simulink model "NeuromuscularModelwReflex2"  (R2019b)
settings: Solver=ode15s  StartTime=0.0  StopTime=30  MaxStep=.01  RelTol=1e-4  AbsTol=1e-6  EnableMultiTasking=on
values from neighbouring files (symbols this model uses):
  dt_visual = 1/30    (= 0.0333333333333)    [evaluateCost.m]    (also in optimize.m)
  LceOffsetTA = 1-0.5*w    [ControlParams.m]
  legAngleTgt = 1.2    [ControlParams.m]    (also in assignGains_novirtmuscle.m = Gains(38))
  LlegLengthClr = .9    (= 0.9)    [ControlParams.m]    (also in assignGains.m = Gains(39); assignGains_novirtmuscle.m = Gains(20))
  LongDelay = 0.020    (= 0.02)    [ControlParams.m]
  MidDelay = 0.010    (= 0.01)    [ControlParams.m]
  RlegLengthClr = .9    (= 0.9)    [ControlParams.m]    (also in assignGains.m = Gains(83); assignGains_novirtmuscle.m = Gains(34))
  ShortDelay = 0.005    [ControlParams.m]
  simbiconGainD = 5*pi/180    (= 0.0872664625997)    [ControlParams.m]    (also in assignGains_novirtmuscle.m = Gains(35))
  simbiconGainV = 5*pi/180    (= 0.0872664625997)    [ControlParams.m]    (also in assignGains_novirtmuscle.m = Gains(36))
  simbiconLegAngle0 = 85*pi/180    (= 1.4835298642)    [ControlParams.m]    (also in assignGains_novirtmuscle.m = Gains(37))
  termination_height = 0.5    [ControlParams.m]
undefined symbols (not defined in the file or in its folder): footCenterToCGDist, footInertia, footMass, g, loptGAS, loptHAM, loptHAMCut, loptTA, lslackGAS, lslackHAM, lslackHAMCut, phimaxGASa, phimaxGASk, phimaxHAMk, phirefGASa, phirefGASk, phirefHAMh, phirefHAMk, rGASa, rGASk, rHAMh, rHAMk, rhoGASa, rhoGASk, rhoHAMh, rhoHAMk, X, Y, Z
libraries: NeuroMuscularLibrary x88, sm_lib x22, nesl_utility x20, simulink x6, simulink_extras x2
(part 3 of 3)

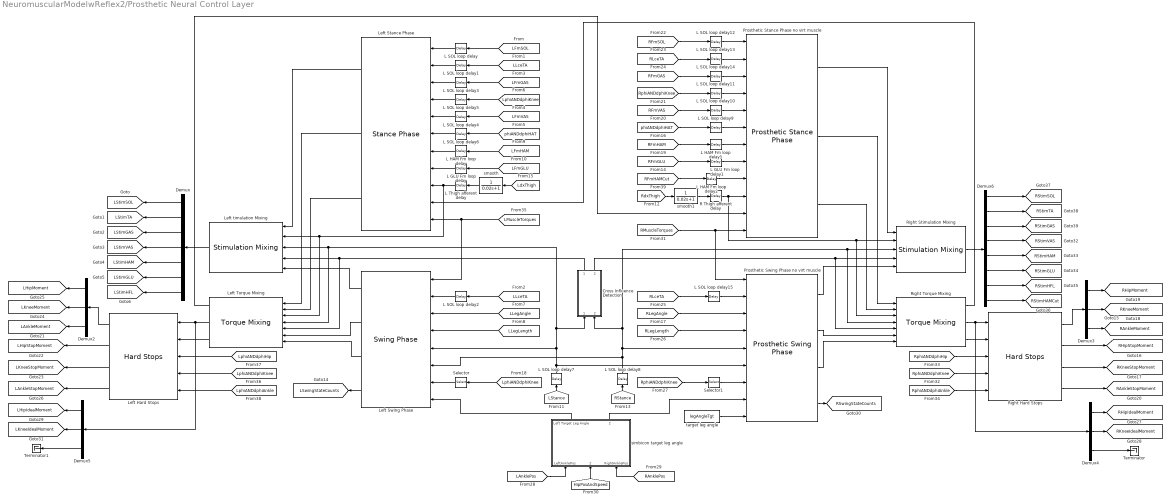
== system NeuromuscularModelwReflex2/Prosthetic Neural Control Layer ==
  Cross Influence Detection : Subsystem
  Demux : Demux  Outputs=7
  Demux{2..5} (4 alike) : Demux  Outputs=3
  Demux6 : Demux  Outputs=8
  L GLU Fm loop delay : TransportDelay  DelayTime=ShortDelay
  L GLU Fm loop delay1 : TransportDelay  DelayTime=ShortDelay
  L HAM Fm loop delay : TransportDelay  DelayTime=ShortDelay
  L HAM Fm loop delay1 : TransportDelay  DelayTime=ShortDelay
  L HAM Fm loop delay2 : TransportDelay  DelayTime=ShortDelay  BufferSize=2048
  L SOL loop delay{,1..3,12..15} (8 alike) : TransportDelay  DelayTime=LongDelay
  L SOL loop delay{4..5,7..8,10..11} (6 alike) : TransportDelay  DelayTime=MidDelay
  L SOL loop delay6 : TransportDelay  DelayTime=ShortDelay
  L SOL loop delay9 : TransportDelay  DelayTime=ShortDelay
  L Thigh afferent delay : TransportDelay  DelayTime=ShortDelay
  Left Hard Stops : NeuroMuscularLibrary/Hard Stops  SystemSampleTime=-1  Latency=0  AutoFrameSizeCalculation=off
  Left Stance Phase : NeuroMuscularLibrary/Stance Phase  GainHAM=LGainHAM  GainGLU=LGainGLU  GainSOL=LGainSOL  GainSOLTA=LGainSOLTA  GainTA=LGainTA  GainGAS=LGainGAS  GainVAS=LGainVAS  GainKneeOverExt=LGainKneeOverExt  PosGainGG=LPosGainGG  SpeedGainGG=LSpeedGainGG  Kglu=LKglu
  Left Swing Phase : NeuroMuscularLibrary/Swing Phase  GainTA=LGainTA  hipPGain=LhipPGain  hipDGain=LhipDGain  legAngleFilter=LlegAngleFilter  kneeFlexGain=LkneeFlexGain  kneeHoldGain1=LkneeHoldGain1  kneeHoldGain2=LkneeHoldGain2  kneeStopGain=LkneeStopGain  kneeExtendGain=LkneeExtendGain  legLengthClr=LlegLengthClr
  Left Torque Mixing : NeuroMuscularLibrary/Torque Mixing  SystemSampleTime=-1  Latency=0  AutoFrameSizeCalculation=off
  Left timulation Mixing : NeuroMuscularLibrary/Stimulation Mixing  SystemSampleTime=-1  Latency=0  AutoFrameSizeCalculation=off
  Prosthetic Stance Phase no virt muscle : NeuroMuscularLibrary/Prosthetic Stance Phase  GainHAM=RGainHAM  GainHAMCut=RGainHAMCut  GainGLU=RGainGLU  GainSOL=RGainSOL  GainSOLTA=RGainSOLTA  GainTA=RGainTA  GainGAS=RGainGAS  GainVAS=RGainVAS  GainKneeOverExt=RGainKneeOverExt  PosGainGG=RPosGainGG  SpeedGainGG=RSpeedGainGG  Kglu=RKglu
  Prosthetic Swing Phase no virt muscle : NeuroMuscularLibrary/Prosthetic Swing Phase  GainTA=RGainTA  hipPGain=RhipPGain  hipDGain=RhipDGain  legAngleFilter=RlegAngleFilter  kneeFlexGain=RkneeFlexGain  kneeHoldGain1=RkneeHoldGain1  kneeHoldGain2=RkneeHoldGain2  kneeStopGain=RkneeStopGain  kneeExtendGain=RkneeExtendGain  legLengthClr=RlegLengthClr
  R Thigh afferent delay : TransportDelay  DelayTime=ShortDelay
  Right Hard Stops : NeuroMuscularLibrary/Hard Stops  SystemSampleTime=-1  Latency=0  AutoFrameSizeCalculation=off
  Right Stimulation Mixing : NeuroMuscularLibrary/Stimulation Mixing  SystemSampleTime=-1  Latency=0  AutoFrameSizeCalculation=off
  Right Torque Mixing : NeuroMuscularLibrary/Torque Mixing  SystemSampleTime=-1  Latency=0  AutoFrameSizeCalculation=off
  Selector : Selector  InputPortWidth=2  IndexOptions=Index vector (dialog)  Indices=2  OutputSizes=1
  Selector1 : Selector  InputPortWidth=2  IndexOptions=Index vector (dialog)  Indices=2  OutputSizes=1
  Terminator : Terminator
  Terminator1 : Terminator
  simbicon target leg angle : Subsystem
  smooth : TransferFcn  Denominator=[0.02 1]
  smooth1 : TransferFcn  Denominator=[0.02 1]
  target leg angle : Constant  Value=legAngleTgt
  tag scope: LAnkleMoment=global, LAnkleStopMoment=global, LHipIdealMoment=global, LHipMoment=global, LHipStopMoment=global, LKneeIdealMoment=global, LKneeMoment=global, LKneeStopMoment=global, LStimGAS=global, LStimGLU=global, LStimHAM=global, LStimHFL=global, LStimSOL=global, LStimTA=global, LStimVAS=global, LSwingStateCounts=global, RAnkleMoment=global, RAnkleStopMoment=global, RHipIdealMoment=global, RHipMoment=global, RHipStopMoment=global, RKneeIdealMoment=global, RKneeMoment=global, RKneeStopMoment=global, RStimGAS=global, RStimGLU=global, RStimHAM=global, RStimHAMCut=global, RStimHFL=global, RStimSOL=global, RStimTA=global, RStimVAS=global, RSwingStateCounts=global
  wires:
  [LFmSOL] -> L SOL loop delay/1
  L SOL loop delay/1 -> Left Stance Phase/1
  [LLceTA] -> L SOL loop delay1/1
  L SOL loop delay1/1 -> Left Stance Phase/2
  Demux/1 -> [LStimSOL]
  Demux/2 -> [LStimTA]
  Demux/3 -> [LStimGAS]
  [LFmGAS] -> L SOL loop delay3/1
  L SOL loop delay3/1 -> Left Stance Phase/3
  [LLceTA] -> L SOL loop delay2/1
  L SOL loop delay4/1 -> Left Stance Phase/5
  [LFmVAS] -> L SOL loop delay4/1
  L SOL loop delay5/1 -> Left Stance Phase/4
  [LphiANDdphiKnee] -> L SOL loop delay5/1
  Demux/4 -> [LStimVAS]
  [phiANDdphiHAT] -> L SOL loop delay6/1
  L SOL loop delay6/1 -> Left Stance Phase/6
  Demux/5 -> [LStimHAM]
  Demux/6 -> [LStimGLU]
  Demux/7 -> [LStimHFL]
  [LdxThigh] -> smooth/1
  smooth/1 -> L Thigh afferent delay/1
  [RdxThigh] -> smooth1/1
  smooth1/1 -> R Thigh afferent delay/1
  [LFmHAM] -> L HAM Fm loop delay/1
  [LFmGLU] -> L GLU Fm loop delay/1
  L SOL loop delay7/1 -> Prosthetic Swing Phase no virt muscle/6, Left Swing Phase/5, Left Torque Mixing/4, Left timulation Mixing/3, Cross Influence Detection/1(LStance)
  [RFmHAM] -> L HAM Fm loop delay1/1
  [RFmGLU] -> L GLU Fm loop delay1/1
  [phiANDdphiHAT] -> L SOL loop delay9/1
  L SOL loop delay9/1 -> Prosthetic Stance Phase no virt muscle/6
  [LStance] -> L SOL loop delay7/1
  [RStance] -> L SOL loop delay8/1
  [RFmVAS] -> L SOL loop delay10/1
  [RphiANDdphiKnee] -> L SOL loop delay11/1
  L SOL loop delay10/1 -> Prosthetic Stance Phase no virt muscle/5
  L SOL loop delay11/1 -> Prosthetic Stance Phase no virt muscle/4
  L SOL loop delay12/1 -> Prosthetic Stance Phase no virt muscle/1
  [RFmSOL] -> L SOL loop delay12/1
  [RLceTA] -> L SOL loop delay13/1
  L SOL loop delay13/1 -> Prosthetic Stance Phase no virt muscle/2
  [RFmGAS] -> L SOL loop delay14/1
  L SOL loop delay14/1 -> Prosthetic Stance Phase no virt muscle/3
  [RLceTA] -> L SOL loop delay15/1
  L Thigh afferent delay/1 -> Left Torque Mixing/3, Left timulation Mixing/2, Left Stance Phase/9
  L HAM Fm loop delay/1 -> Left Stance Phase/7
  L GLU Fm loop delay/1 -> Left Stance Phase/8
  R Thigh afferent delay/1 -> Prosthetic Stance Phase no virt muscle/10, Right Torque Mixing/3, Right Stimulation Mixing/2
  L SOL loop delay15/1 -> Prosthetic Swing Phase no virt muscle/2
  L SOL loop delay2/1 -> Left Swing Phase/2
  Prosthetic Stance Phase no virt muscle/1 -> Right Stimulation Mixing/1
  L SOL loop delay8/1 -> Left Swing Phase/6, Prosthetic Swing Phase no virt muscle/5, Right Torque Mixing/4, Right Stimulation Mixing/3, Cross Influence Detection/2(RStance)
  Cross Influence Detection/2(LeftLeading) -> Right Torque Mixing/5, Right Stimulation Mixing/4
  Left timulation Mixing/1 -> Demux/1
  Left Stance Phase/1 -> Left timulation Mixing/1
  Cross Influence Detection/1(RightLeading) -> Left Torque Mixing/5, Left timulation Mixing/4
  Demux3/1 -> [RHipMoment]
  Demux3/2 -> [RKneeMoment]
  [LLegAngle] -> Left Swing Phase/3
  [LLegLength] -> Left Swing Phase/4
  [RLegAngle] -> Prosthetic Swing Phase no virt muscle/3
  [RLegLength] -> Prosthetic Swing Phase no virt muscle/4
  [RphiANDdphiKnee] -> Selector1/1
  Selector1/1 -> Prosthetic Swing Phase no virt muscle/7
  [LAnklePos] -> simbicon target leg angle/1(LeftAnklePos)
  [RAnklePos] -> simbicon target leg angle/3(RightAnklePos)
  Prosthetic Swing Phase no virt muscle/1 -> Right Stimulation Mixing/5
  [LphiANDdphiKnee] -> Selector/1
  Selector/1 -> Left Swing Phase/7
  Left Swing Phase/1 -> Left timulation Mixing/5
  [HipPosAndSpeed] -> simbicon target leg angle/2(HIPposAndSpeed)
  simbicon target leg angle/1(Left Target Leg Angle) -> Left Swing Phase/8
  Prosthetic Swing Phase no virt muscle/4 -> [RSwingStateCounts]
  Left Swing Phase/4 -> [LSwingStateCounts]
  Demux3/3 -> [RAnkleMoment]
  [RphiANDdphiKnee] -> Right Hard Stops/4
  [RphiANDdphiHip] -> Right Hard Stops/3
  [RphiANDdphiAnkle] -> Right Hard Stops/5
  Right Hard Stops/2 -> [RHipStopMoment]
  Right Hard Stops/3 -> [RKneeStopMoment]
  Right Hard Stops/4 -> [RAnkleStopMoment]
  [LMuscleTorques] -> Left Swing Phase/1, Left Stance Phase/11
  Demux2/1 -> [LHipMoment]
  Demux2/3 -> [LAnkleMoment]
  Left Hard Stops/1 -> Demux2/1
  [LphiANDdphiKnee] -> Left Hard Stops/4
  [LphiANDdphiHip] -> Left Hard Stops/3
  Left Hard Stops/2 -> [LHipStopMoment]
  Left Hard Stops/3 -> [LKneeStopMoment]
  Left Hard Stops/4 -> [LAnkleStopMoment]
  Left Stance Phase/2 -> Left Torque Mixing/1
  Demux2/2 -> [LKneeMoment]
  Right Torque Mixing/2 -> Demux4/1, Right Hard Stops/1
  Right Hard Stops/1 -> Demux3/1
  [RMuscleTorques] -> Prosthetic Swing Phase no virt muscle/1, Prosthetic Stance Phase no virt muscle/12
  Demux4/1 -> [RHipIdealMoment]
  Demux4/2 -> [RKneeIdealMoment]
  Demux4/3 -> Terminator/1
  Prosthetic Swing Phase no virt muscle/3 -> Right Torque Mixing/7
  Prosthetic Swing Phase no virt muscle/2 -> Right Torque Mixing/6
  Prosthetic Stance Phase no virt muscle/3 -> Right Torque Mixing/2
  Prosthetic Stance Phase no virt muscle/2 -> Right Torque Mixing/1
  Right Torque Mixing/3 -> Right Hard Stops/2
  Right Torque Mixing/1 -> Left Stance Phase/10
  [LphiANDdphiAnkle] -> Left Hard Stops/5
  Left Torque Mixing/2 -> Demux5/1, Left Hard Stops/1
  Left Torque Mixing/3 -> Left Hard Stops/2
  Left Torque Mixing/1 -> Prosthetic Stance Phase no virt muscle/11
  Left Stance Phase/3 -> Left Torque Mixing/2
  Left Swing Phase/2 -> Left Torque Mixing/6
  Left Swing Phase/3 -> Left Torque Mixing/7
  Demux5/1 -> [LHipIdealMoment]
  Demux5/2 -> [LKneeIdealMoment]
  Demux5/3 -> Terminator1/1
  Demux6/1 -> [RStimSOL]
  Demux6/2 -> [RStimTA]
  Demux6/4 -> [RStimVAS]
  Demux6/5 -> [RStimHAM]
  Demux6/7 -> [RStimHFL]
  Demux6/3 -> [RStimGAS]
  Demux6/6 -> [RStimGLU]
  Right Stimulation Mixing/1 -> Demux6/1
  Demux6/8 -> [RStimHAMCut]
  L HAM Fm loop delay1/1 -> Prosthetic Stance Phase no virt muscle/7
  L GLU Fm loop delay1/1 -> Prosthetic Stance Phase no virt muscle/8
  [RFmHAMCut] -> L HAM Fm loop delay2/1
  L HAM Fm loop delay2/1 -> Prosthetic Stance Phase no virt muscle/9
  simbicon target leg angle/2(Right Target Leg Angle) -> Prosthetic Swing Phase no virt muscle/8
  target leg angle/1 -> Prosthetic Swing Phase no virt muscle/9

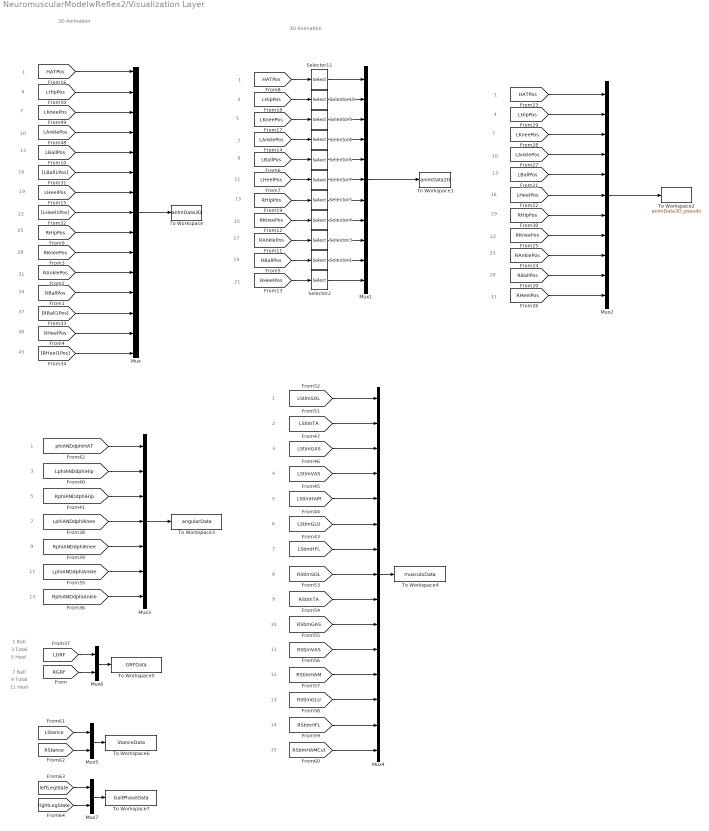
== system NeuromuscularModelwReflex2/Visualization Layer ==
  note: 31
  note: 28
  note: 25
  note: 22
  note: 19
  note: 16
  note: 13
  note: 10
  note: 7
  note: 4
  note: 1
  note: 3D Animation
  note: 21
  note: 17
  note: 11
  note: 7
  note: 15
  note: 9
  note: 3
  note: 1
  note: 13
  note: 3D Animation
  note: 19
  note: 5
  note: 28
  note: 22
  note: 19
  note: 16
  note: 10
  note: 7
  note: 1
  note: 4
  note: 13
  note: 31
  note: 25
  note: 34
  note: 37
  note: 40
  note: 43
  note: 1
  note: 3
  note: 5
  note: 7
  note: 9
  note: 11
  note: 13
  note: 1
  note: 2
  note: 3
  note: 4
  note: 5
  note: 6
  note: 7
  note: 8
  note: 9
  note: 10
  note: 11
  note: 12
  note: 13
  note: 14
  note: 15
  note: 1 Ball
  note: 3 Total
  note: 5 Heel
  note: 7 Ball
  note: 9 Total
  note: 11 Heel
  Mux : Mux  Inputs=15
  Mux1 : Mux  Inputs=11
  Mux2 : Mux  Inputs=11
  Mux3 : Mux  Inputs=7
  Mux4 : Mux  Inputs=15
  Mux5 : Mux  Inputs=2
  Mux6 : Mux  Inputs=2
  Mux7 : Mux  Inputs=2
  Selector{1..11} (11 alike) : Selector  InputPortWidth=3  IndexOptions=Index vector (dialog)  Indices=[1 3]  OutputSizes=1
  To Workspace : ToWorkspace  VariableName=animData3D  SaveFormat=Structure With Time  SampleTime=1/30
  To Workspace1 : ToWorkspace  VariableName=animData2D  SaveFormat=Structure With Time  SampleTime=1/30
  To Workspace2 : ToWorkspace  VariableName=animData3D_pseudo  SaveFormat=Structure With Time  SampleTime=1/30
  To Workspace3 : ToWorkspace  VariableName=angularData  SaveFormat=Structure With Time  SampleTime=1/30
  To Workspace4 : ToWorkspace  VariableName=musculoData  SaveFormat=Structure With Time  SampleTime=1/30
  To Workspace5 : ToWorkspace  VariableName=GRFData  SaveFormat=Structure With Time  SampleTime=1/30
  To Workspace6 : ToWorkspace  VariableName=StanceData  SaveFormat=Structure With Time  SampleTime=1/30
  To Workspace7 : ToWorkspace  VariableName=GaitPhaseData  SaveFormat=Structure With Time  SampleTime=1/30
  wires:
  [HATPos] -> Mux/1
  [LBallPos] -> Mux/5
  [LAnklePos] -> Mux/4
  [LKneePos] -> Mux/3
  [LHipPos] -> Mux/2
  Mux/1 -> To Workspace/1
  [LHeelPos] -> Selector7/1
  Selector3/1 -> Mux1/9
  Selector1/1 -> Mux1/10
  Selector6/1 -> Mux1/5
  Selector2/1 -> Mux1/11
  [LKneePos] -> Selector9/1
  Selector5/1 -> Mux1/7
  Selector4/1 -> Mux1/8
  [LAnklePos] -> Selector8/1
  Selector8/1 -> Mux1/4
  Selector9/1 -> Mux1/3
  [LHipPos] -> Selector10/1
  Selector7/1 -> Mux1/6
  [LBallPos] -> Selector6/1
  Selector10/1 -> Mux1/2
  [HATPos] -> Selector11/1
  [RHipPos] -> Selector5/1
  [RHeelPos] -> Selector2/1
  [RAnklePos] -> Selector3/1
  Mux1/1 -> To Workspace1/1
  [RBallPos] -> Selector1/1
  [RKneePos] -> Selector4/1
  Selector11/1 -> Mux1/1
  [RKneePos] -> Mux2/8
  [RHipPos] -> Mux2/7
  Mux2/1 -> To Workspace2/1
  [RAnklePos] -> Mux2/9
  [LAnklePos] -> Mux2/4
  [LHipPos] -> Mux2/2
  [LHeelPos] -> Mux2/6
  [LKneePos] -> Mux2/3
  [RHeelPos] -> Mux2/11
  [HATPos] -> Mux2/1
  [LBallPos] -> Mux2/5
  [RBallPos] -> Mux2/10
  [LBall1Pos] -> Mux/6
  [LHeelPos] -> Mux/7
  [LHeel1Pos] -> Mux/8
  [RHipPos] -> Mux/9
  [RKneePos] -> Mux/10
  [RAnklePos] -> Mux/11
  [RBallPos] -> Mux/12
  [RBall1Pos] -> Mux/13
  [RHeelPos] -> Mux/14
  [RHeel1Pos] -> Mux/15
  [phiANDdphiHAT] -> Mux3/1
  [LphiANDdphiHip] -> Mux3/2
  [RphiANDdphiHip] -> Mux3/3
  [LphiANDdphiKnee] -> Mux3/4
  [RphiANDdphiKnee] -> Mux3/5
  [LphiANDdphiAnkle] -> Mux3/6
  [RphiANDdphiAnkle] -> Mux3/7
  [LStimSOL] -> Mux4/1
  [LStimTA] -> Mux4/2
  [LStimGAS] -> Mux4/3
  [LStimVAS] -> Mux4/4
  [LStimHAM] -> Mux4/5
  [LStimGLU] -> Mux4/6
  [LStimHFL] -> Mux4/7
  [RStimSOL] -> Mux4/8
  [RStimTA] -> Mux4/9
  [RStimGAS] -> Mux4/10
  [RStimVAS] -> Mux4/11
  [RStimHAM] -> Mux4/12
  [RStimGLU] -> Mux4/13
  [RStimHFL] -> Mux4/14
  [RStimHAMCut] -> Mux4/15
  [LGRF] -> Mux6/1
  Mux3/1 -> To Workspace3/1
  Mux4/1 -> To Workspace4/1
  Mux6/1 -> To Workspace5/1
  [RGRF] -> Mux6/2
  [RStance] -> Mux5/2
  Mux5/1 -> To Workspace6/1
  [LStance] -> Mux5/1
  [leftLegState] -> Mux7/1
  Mux7/1 -> To Workspace7/1
  [rightLegState] -> Mux7/2

== system NeuromuscularModelwReflex2/Prosthetic Body Mechanics Layer/HAT Speed Sensor ==
  PS-Simulink Converter1 : nesl_utility/PS-Simulink Converter  PhysicalDomain=network_engine_domain  SubClassName=ps_output  LeftPortType=input  RightPortType=output  PseudoPeriodic=off  Frequencies=[]  Unit=m/s  AffineConversion=off
  Position Sensor : sm_lib/Frames and Transforms/Transform Sensor  MeasurementFrame=World  SenseAngle=off  SenseAxis=off  SenseAngle1=off  SenseAngle2=off  SenseAngle3=off  SenseQ=off  SenseR=off  SenseOmegaX=off  SenseOmegaY=off  SenseOmegaZ=off  SenseOmega1=off  SenseOmega2=off  SenseOmega3=off  SenseQDot=off  SenseRDot=off  SenseAlphaX=off  SenseAlphaY=off  SenseAlphaZ=off  SenseAlpha1=off  SenseAlpha2=off  SenseAlpha3=off  SenseQDDot=off  SenseRDDot=off  SenseX=off  SenseY=off  SenseZ=off  SenseRad=off  SenseAzim=off  SenseDist=off  SenseInc=off  SenseXDot=on  SenseYDot=off  SenseZDot=off  SenseRadDot=off  SenseAzimDot=off  SenseDistDot=off  SenseIncDot=off  SenseXDDot=off  SenseYDDot=off  SenseZDDot=off  SenseRadDDot=off  SenseAzimDDot=off  SenseDistDDot=off  SenseIncDDot=off
  World Frame : sm_lib/Frames and Transforms/World Frame
  Frame : PMIOPort  Side=Left
  Speed : Outport
  wires:
  PS-Simulink Converter1/1 -> Speed/1
  connections:
  Position Sensor/LConn1 -- World Frame/RConn1
  Position Sensor/RConn1 -- Frame/RConn1
  Position Sensor/RConn2 -- PS-Simulink Converter1/LConn1

== system NeuromuscularModelwReflex2/Prosthetic Body Mechanics Layer/Hip Pos//Speed Sensor ==
  Mux : Mux  Inputs=3
  PS-Simulink Converter : nesl_utility/PS-Simulink Converter  PhysicalDomain=network_engine_domain  SubClassName=ps_output  LeftPortType=input  RightPortType=output  PseudoPeriodic=off  Frequencies=[]  Unit=m  AffineConversion=off
  PS-Simulink Converter1 : nesl_utility/PS-Simulink Converter  PhysicalDomain=network_engine_domain  SubClassName=ps_output  LeftPortType=input  RightPortType=output  PseudoPeriodic=off  Frequencies=[]  Unit=m  AffineConversion=off
  PS-Simulink Converter2 : nesl_utility/PS-Simulink Converter  PhysicalDomain=network_engine_domain  SubClassName=ps_output  LeftPortType=input  RightPortType=output  PseudoPeriodic=off  Frequencies=[]  Unit=m/s  AffineConversion=off
  Position Sensor : sm_lib/Frames and Transforms/Transform Sensor  MeasurementFrame=World  SenseAngle=off  SenseAxis=off  SenseAngle1=off  SenseAngle2=off  SenseAngle3=off  SenseQ=off  SenseR=off  SenseOmegaX=off  SenseOmegaY=off  SenseOmegaZ=off  SenseOmega1=off  SenseOmega2=off  SenseOmega3=off  SenseQDot=off  SenseRDot=off  SenseAlphaX=off  SenseAlphaY=off  SenseAlphaZ=off  SenseAlpha1=off  SenseAlpha2=off  SenseAlpha3=off  SenseQDDot=off  SenseRDDot=off  SenseX=on  SenseY=off  SenseZ=on  SenseRad=off  SenseAzim=off  SenseDist=off  SenseInc=off  SenseXDot=on  SenseYDot=off  SenseZDot=off  SenseRadDot=off  SenseAzimDot=off  SenseDistDot=off  SenseIncDot=off  SenseXDDot=off  SenseYDDot=off  SenseZDDot=off  SenseRadDDot=off  SenseAzimDDot=off  SenseDistDDot=off  SenseIncDDot=off
  World Frame : sm_lib/Frames and Transforms/World Frame
  Frame : PMIOPort  Side=Left
  PosSpeed : Outport
  wires:
  Mux/1 -> PosSpeed/1
  PS-Simulink Converter/1 -> Mux/1
  PS-Simulink Converter1/1 -> Mux/2
  PS-Simulink Converter2/1 -> Mux/3
  connections:
  Position Sensor/LConn1 -- World Frame/RConn1
  Position Sensor/RConn1 -- Frame/RConn1
  PS-Simulink Converter/LConn1 -- Position Sensor/RConn2
  PS-Simulink Converter1/LConn1 -- Position Sensor/RConn3
  PS-Simulink Converter2/LConn1 -- Position Sensor/RConn4

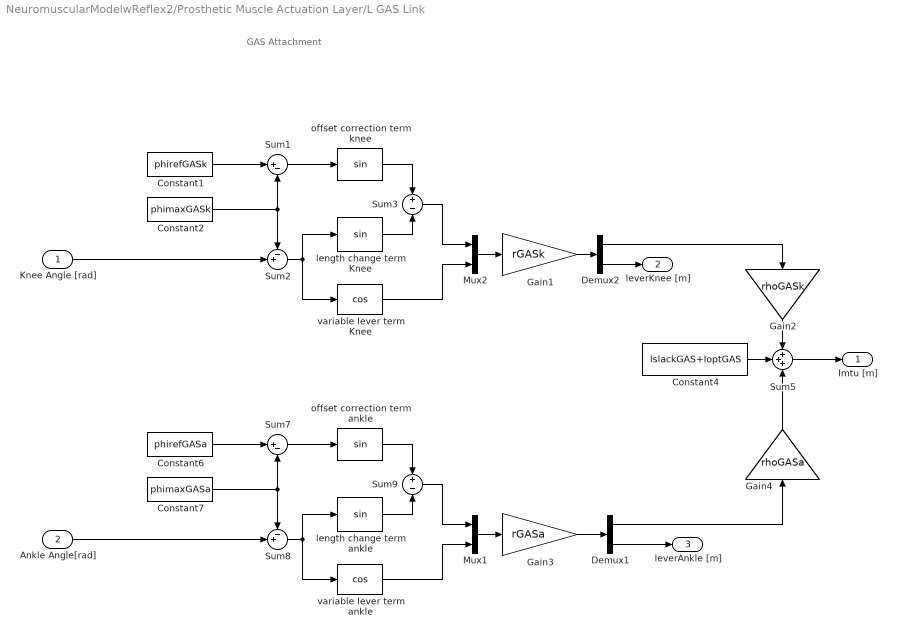
== system NeuromuscularModelwReflex2/Prosthetic Muscle Actuation Layer/L GAS Link ==
  note: GAS Attachment
  Knee Angle [rad] : Inport
  Ankle Angle[rad] : Inport  Port=2
  Constant1 : Constant  Value=phirefGASk
  Constant2 : Constant  Value=phimaxGASk
  Constant4 : Constant  Value=lslackGAS+loptGAS
  Constant6 : Constant  Value=phirefGASa
  Constant7 : Constant  Value=phimaxGASa
  Demux1 : Demux  Outputs=2
  Demux2 : Demux  Outputs=2
  Gain1 : Gain  Gain=rGASk
  Gain2 : Gain  Gain=rhoGASk
  Gain3 : Gain  Gain=rGASa
  Gain4 : Gain  Gain=rhoGASa
  Mux1 : Mux  Inputs=2
  Mux2 : Mux  Inputs=2
  Sum1 : Sum  Inputs=|+-
  Sum2 : Sum  Inputs=-+|
  Sum3 : Sum  Inputs=+-
  Sum5 : Sum  Inputs=+++
  Sum7 : Sum  Inputs=|+-
  Sum8 : Sum  Inputs=-+|
  Sum9 : Sum  Inputs=+-
  length change term Knee : Trigonometry
  length change term ankle : Trigonometry
  offset correction term ankle : Trigonometry
  offset correction term knee : Trigonometry
  variable lever term Knee : Trigonometry  Operator=cos
  variable lever term ankle : Trigonometry  Operator=cos
  lmtu [m] : Outport
  leverKnee [m] : Outport  Port=2
  leverAnkle [m] : Outport  Port=3
  wires:
  Ankle Angle[rad]/1 -> Sum8/2
  Sum5/1 -> lmtu [m]/1
  variable lever term ankle/1 -> Mux1/2
  Demux1/2 -> leverAnkle [m]/1
  Sum8/1 -> variable lever term ankle/1, length change term ankle/1
  Constant7/1 -> Sum8/1, Sum7/2
  Sum7/1 -> offset correction term ankle/1
  Constant6/1 -> Sum7/1
  length change term ankle/1 -> Sum9/2
  offset correction term ankle/1 -> Sum9/1
  Sum9/1 -> Mux1/1
  Constant4/1 -> Sum5/2
  Mux1/1 -> Gain3/1
  Gain3/1 -> Demux1/1
  Demux1/1 -> Gain4/1
  Gain4/1 -> Sum5/3
  Knee Angle [rad]/1 -> Sum2/2
  variable lever term Knee/1 -> Mux2/2
  Sum2/1 -> variable lever term Knee/1, length change term Knee/1
  Constant2/1 -> Sum2/1, Sum1/2
  Sum1/1 -> offset correction term knee/1
  Constant1/1 -> Sum1/1
  length change term Knee/1 -> Sum3/2
  offset correction term knee/1 -> Sum3/1
  Sum3/1 -> Mux2/1
  Mux2/1 -> Gain1/1
  Gain1/1 -> Demux2/1
  Demux2/2 -> leverKnee [m]/1
  Demux2/1 -> Gain2/1
  Gain2/1 -> Sum5/1

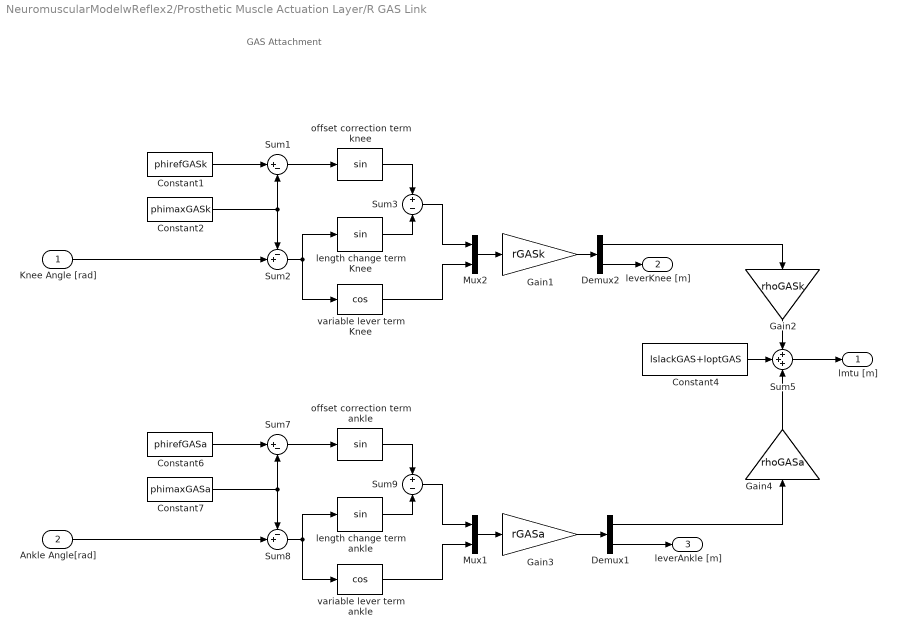
== system NeuromuscularModelwReflex2/Prosthetic Muscle Actuation Layer/R GAS Link ==
  note: GAS Attachment
  Knee Angle [rad] : Inport
  Ankle Angle[rad] : Inport  Port=2
  Constant1 : Constant  Value=phirefGASk
  Constant2 : Constant  Value=phimaxGASk
  Constant4 : Constant  Value=lslackGAS+loptGAS
  Constant6 : Constant  Value=phirefGASa
  Constant7 : Constant  Value=phimaxGASa
  Demux1 : Demux  Outputs=2
  Demux2 : Demux  Outputs=2
  Gain1 : Gain  Gain=rGASk
  Gain2 : Gain  Gain=rhoGASk
  Gain3 : Gain  Gain=rGASa
  Gain4 : Gain  Gain=rhoGASa
  Mux1 : Mux  Inputs=2
  Mux2 : Mux  Inputs=2
  Sum1 : Sum  Inputs=|+-
  Sum2 : Sum  Inputs=-+|
  Sum3 : Sum  Inputs=+-
  Sum5 : Sum  Inputs=+++
  Sum7 : Sum  Inputs=|+-
  Sum8 : Sum  Inputs=-+|
  Sum9 : Sum  Inputs=+-
  length change term Knee : Trigonometry
  length change term ankle : Trigonometry
  offset correction term ankle : Trigonometry
  offset correction term knee : Trigonometry
  variable lever term Knee : Trigonometry  Operator=cos
  variable lever term ankle : Trigonometry  Operator=cos
  lmtu [m] : Outport
  leverKnee [m] : Outport  Port=2
  leverAnkle [m] : Outport  Port=3
  wires:
  Ankle Angle[rad]/1 -> Sum8/2
  Sum5/1 -> lmtu [m]/1
  variable lever term ankle/1 -> Mux1/2
  Demux1/2 -> leverAnkle [m]/1
  Sum8/1 -> variable lever term ankle/1, length change term ankle/1
  Constant7/1 -> Sum8/1, Sum7/2
  Sum7/1 -> offset correction term ankle/1
  Constant6/1 -> Sum7/1
  length change term ankle/1 -> Sum9/2
  offset correction term ankle/1 -> Sum9/1
  Sum9/1 -> Mux1/1
  Constant4/1 -> Sum5/2
  Mux1/1 -> Gain3/1
  Gain3/1 -> Demux1/1
  Demux1/1 -> Gain4/1
  Gain4/1 -> Sum5/3
  Knee Angle [rad]/1 -> Sum2/2
  variable lever term Knee/1 -> Mux2/2
  Sum2/1 -> variable lever term Knee/1, length change term Knee/1
  Constant2/1 -> Sum2/1, Sum1/2
  Sum1/1 -> offset correction term knee/1
  Constant1/1 -> Sum1/1
  length change term Knee/1 -> Sum3/2
  offset correction term knee/1 -> Sum3/1
  Sum3/1 -> Mux2/1
  Mux2/1 -> Gain1/1
  Gain1/1 -> Demux2/1
  Demux2/2 -> leverKnee [m]/1
  Demux2/1 -> Gain2/1
  Gain2/1 -> Sum5/1

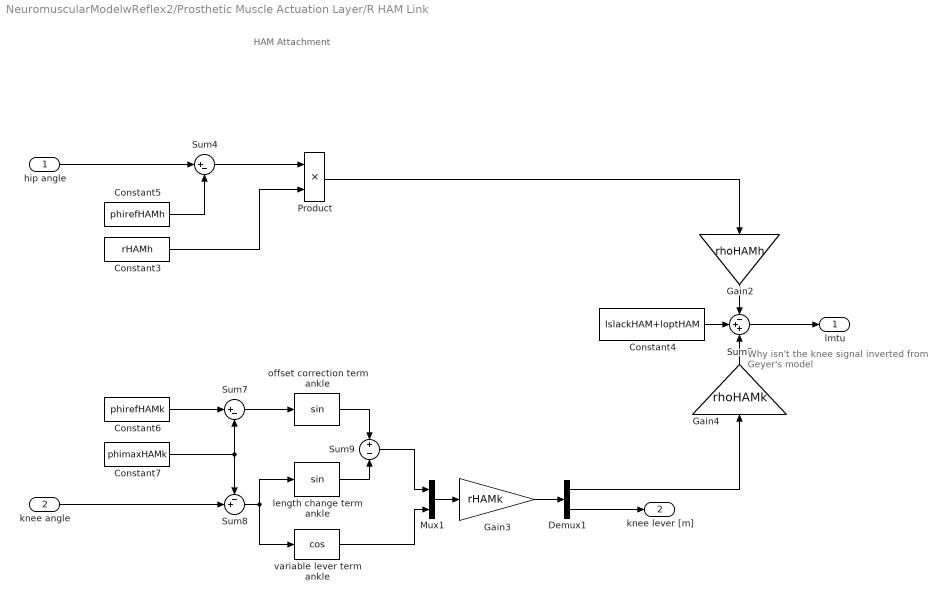
== system NeuromuscularModelwReflex2/Prosthetic Muscle Actuation Layer/R HAM Link ==
  note: HAM Attachment
  note: Why isn't the knee signal inverted from
      | Geyer's model
  hip angle : Inport
  knee angle : Inport  Port=2
  Constant3 : Constant  Value=rHAMh
  Constant4 : Constant  Value=lslackHAM+loptHAM
  Constant5 : Constant  Value=phirefHAMh
  Constant6 : Constant  Value=phirefHAMk
  Constant7 : Constant  Value=phimaxHAMk  VectorParams1D=off
  Demux1 : Demux  Outputs=2
  Gain2 : Gain  Gain=rhoHAMh
  Gain3 : Gain  Gain=rHAMk
  Gain4 : Gain  Gain=rhoHAMk
  Mux1 : Mux  Inputs=2
  Product : Product  RndMeth=Zero
  Sum4 : Sum  Inputs=|+-
  Sum5 : Sum  Inputs=-++
  Sum7 : Sum  Inputs=|+-
  Sum8 : Sum  Inputs=-+|
  Sum9 : Sum  Inputs=+-
  length change term ankle : Trigonometry
  offset correction term ankle : Trigonometry
  variable lever term ankle : Trigonometry  Operator=cos
  lmtu : Outport
  knee lever [m] : Outport  Port=2
  wires:
  knee angle/1 -> Sum8/2
  hip angle/1 -> Sum4/1
  Gain2/1 -> Sum5/1
  Gain4/1 -> Sum5/3
  Demux1/1 -> Gain4/1
  Gain3/1 -> Demux1/1
  Mux1/1 -> Gain3/1
  Constant4/1 -> Sum5/2
  Sum9/1 -> Mux1/1
  offset correction term ankle/1 -> Sum9/1
  length change term ankle/1 -> Sum9/2
  Constant6/1 -> Sum7/1
  Sum7/1 -> offset correction term ankle/1
  Constant7/1 -> Sum7/2, Sum8/1
  Sum8/1 -> length change term ankle/1, variable lever term ankle/1
  Demux1/2 -> knee lever [m]/1
  variable lever term ankle/1 -> Mux1/2
  Sum5/1 -> lmtu/1
  Product/1 -> Gain2/1
  Constant3/1 -> Product/2
  Sum4/1 -> Product/1
  Constant5/1 -> Sum4/2

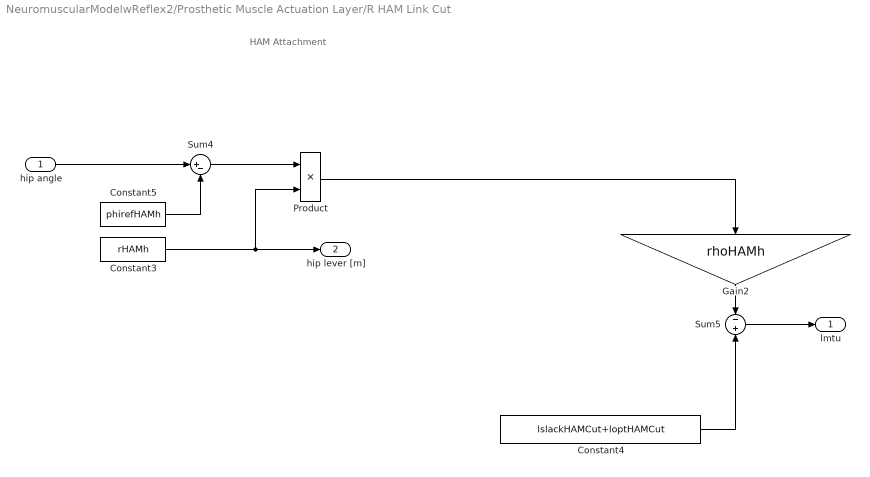
== system NeuromuscularModelwReflex2/Prosthetic Muscle Actuation Layer/R HAM Link Cut ==
  note: HAM Attachment
  hip angle : Inport
  Constant3 : Constant  Value=rHAMh
  Constant4 : Constant  Value=lslackHAMCut+loptHAMCut
  Constant5 : Constant  Value=phirefHAMh
  Gain2 : Gain  Gain=rhoHAMh
  Product : Product  RndMeth=Zero
  Sum4 : Sum  Inputs=|+-
  Sum5 : Sum  Inputs=-+
  lmtu : Outport
  hip lever [m] : Outport  Port=2
  wires:
  hip angle/1 -> Sum4/1
  Gain2/1 -> Sum5/1
  Constant4/1 -> Sum5/2
  Sum5/1 -> lmtu/1
  Product/1 -> Gain2/1
  Constant3/1 -> Product/2, hip lever [m]/1
  Sum4/1 -> Product/1
  Constant5/1 -> Sum4/2

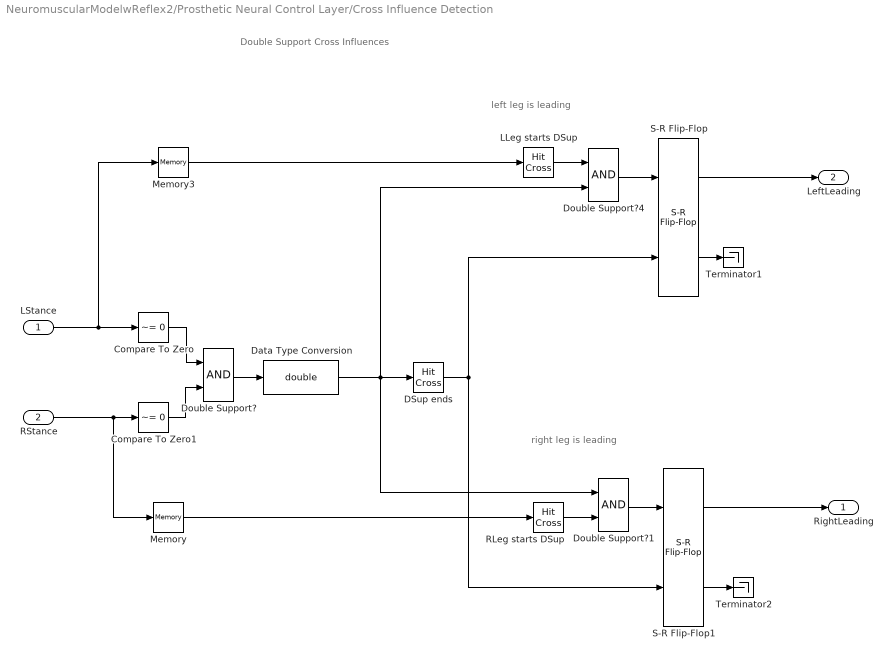
== system NeuromuscularModelwReflex2/Prosthetic Neural Control Layer/Cross Influence Detection ==
  note: right leg is leading
  note: left leg is leading
  note: Double Support Cross Influences
  LStance : Inport
  RStance : Inport  Port=2
  Compare To Zero : simulink/Logic and Bit Operations/Compare To Zero  relop=~=  OutDataTypeStr=boolean
  Compare To Zero1 : simulink/Logic and Bit Operations/Compare To Zero  relop=~=  OutDataTypeStr=boolean
  DSup ends : HitCross  HitCrossingOffset=0.5  HitCrossingDirection=falling  ZeroCross=off
  Data Type Conversion : DataTypeConversion  OutDataTypeStr=double
  Double Support? : Logic  AllPortsSameDT=off
  Double Support?1 : Logic  AllPortsSameDT=off
  Double Support?4 : Logic  AllPortsSameDT=off
  LLeg starts DSup : HitCross  HitCrossingOffset=0.5  HitCrossingDirection=rising  ZeroCross=off
  Memory : Memory
  Memory3 : Memory
  RLeg starts DSup : HitCross  HitCrossingOffset=0.5  HitCrossingDirection=rising  ZeroCross=off
  S-R Flip-Flop : simulink_extras/Flip Flops/S-R Flip-Flop  initial_condition=0
  S-R Flip-Flop1 : simulink_extras/Flip Flops/S-R Flip-Flop  initial_condition=0
  Terminator1 : Terminator
  Terminator2 : Terminator
  RightLeading : Outport
  LeftLeading : Outport  Port=2
  wires:
  S-R Flip-Flop/2 -> Terminator1/1
  S-R Flip-Flop/1 -> LeftLeading/1
  S-R Flip-Flop1/2 -> Terminator2/1
  LStance/1 -> Memory3/1, Compare To Zero/1
  RStance/1 -> Compare To Zero1/1, Memory/1
  S-R Flip-Flop1/1 -> RightLeading/1
  Memory/1 -> RLeg starts DSup/1
  RLeg starts DSup/1 -> Double Support?1/2
  Double Support?1/1 -> S-R Flip-Flop1/1
  Memory3/1 -> LLeg starts DSup/1
  LLeg starts DSup/1 -> Double Support?4/1
  Double Support?4/1 -> S-R Flip-Flop/1
  DSup ends/1 -> S-R Flip-Flop/2, S-R Flip-Flop1/2
  Compare To Zero/1 -> Double Support?/1
  Compare To Zero1/1 -> Double Support?/2
  Double Support?/1 -> Data Type Conversion/1
  Data Type Conversion/1 -> Double Support?1/1, Double Support?4/2, DSup ends/1

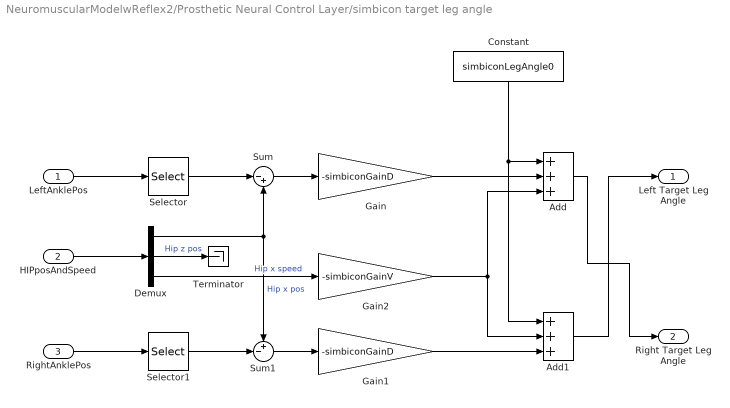
== system NeuromuscularModelwReflex2/Prosthetic Neural Control Layer/simbicon target leg angle ==
  LeftAnklePos : Inport
  HIPposAndSpeed : Inport  Port=2
  RightAnklePos : Inport  Port=3
  Add : Sum  Inputs=+++
  Add1 : Sum  Inputs=+++
  Constant : Constant  Value=simbiconLegAngle0
  Demux : Demux  Outputs=3
  Gain : Gain  Gain=-simbiconGainD
  Gain1 : Gain  Gain=-simbiconGainD
  Gain2 : Gain  Gain=-simbiconGainV
  Selector : Selector  InputPortWidth=3  IndexOptions=Index vector (dialog)  Indices=[1]  OutputSizes=1
  Selector1 : Selector  InputPortWidth=3  IndexOptions=Index vector (dialog)  Indices=[1]  OutputSizes=1
  Sum : Sum  Inputs=|-+
  Sum1 : Sum  Inputs=+-|
  Terminator : Terminator
  Left Target Leg Angle : Outport
  Right Target Leg Angle : Outport  Port=2
  wires:
  HIPposAndSpeed/1 -> Demux/1
  Demux/1 -> Sum1/1, Sum/2  "Hip x pos"
  Sum/1 -> Gain/1
  Sum1/1 -> Gain1/1
  Gain/1 -> Add/2
  Gain2/1 -> Add/3, Add1/2
  Gain1/1 -> Add1/3
  Constant/1 -> Add/1, Add1/1
  Add1/1 -> Left Target Leg Angle/1
  Add/1 -> Right Target Leg Angle/1
  LeftAnklePos/1 -> Selector/1
  Selector/1 -> Sum/1
  RightAnklePos/1 -> Selector1/1
  Selector1/1 -> Sum1/2
  Demux/3 -> Gain2/1  "Hip x speed"
  Demux/2 -> Terminator/1  "Hip z pos"
